simulink model "ProcessNetworkSimulation"  (R2015b)
settings: Solver=VariableStepAuto  StartTime=0.0  StopTime=1000.0  RelTol=1e-3
libraries: simulink x1, simeventslib x1
(part 8 of 21)

== system ProcessNetworkSimulation/Process_4 ==
  IN_Job : PathCombiner  NumberInputPorts=42
  OUT_Job : OutputSwitch  NumberOutputPorts=37  SwitchingCriterion=From attribute  AttributeName=outputFlowNode
  Process : Subsystem
  IN_Job_1 : PMIOPort  Port=1  Side=Left
  IN_Job_2 : PMIOPort  Port=2  Side=Left
  IN_Job_3 : PMIOPort  Port=3  Side=Left
  IN_Job_4 : PMIOPort  Port=4  Side=Left
  IN_Job_5 : PMIOPort  Port=5  Side=Left
  IN_Job_6 : PMIOPort  Port=6  Side=Left
  IN_Job_7 : PMIOPort  Port=7  Side=Left
  IN_Job_8 : PMIOPort  Port=8  Side=Left
  IN_Job_9 : PMIOPort  Port=9  Side=Left
  IN_Job_10 : PMIOPort  Port=10  Side=Left
  IN_Job_11 : PMIOPort  Port=11  Side=Left
  IN_Job_12 : PMIOPort  Port=12  Side=Left
  IN_Job_13 : PMIOPort  Port=13  Side=Left
  IN_Job_14 : PMIOPort  Port=14  Side=Left
  IN_Job_15 : PMIOPort  Port=15  Side=Left
  IN_Job_16 : PMIOPort  Port=16  Side=Left
  IN_Job_17 : PMIOPort  Port=17  Side=Left
  IN_Job_18 : PMIOPort  Port=18  Side=Left
  IN_Job_19 : PMIOPort  Port=19  Side=Left
  IN_Job_20 : PMIOPort  Port=20  Side=Left
  IN_Job_21 : PMIOPort  Port=21  Side=Left
  IN_Job_22 : PMIOPort  Port=22  Side=Left
  IN_Job_23 : PMIOPort  Port=23  Side=Left
  IN_Job_24 : PMIOPort  Port=24  Side=Left
  IN_Job_25 : PMIOPort  Port=25  Side=Left
  IN_Job_26 : PMIOPort  Port=26  Side=Left
  IN_Job_27 : PMIOPort  Port=27  Side=Left
  IN_Job_28 : PMIOPort  Port=28  Side=Left
  IN_Job_29 : PMIOPort  Port=29  Side=Left
  IN_Job_30 : PMIOPort  Port=30  Side=Left
  IN_Job_31 : PMIOPort  Port=31  Side=Left
  IN_Job_32 : PMIOPort  Port=32  Side=Left
  IN_Job_33 : PMIOPort  Port=33  Side=Left
  IN_Job_34 : PMIOPort  Port=34  Side=Left
  IN_Job_35 : PMIOPort  Port=35  Side=Left
  IN_Job_36 : PMIOPort  Port=36  Side=Left
  IN_Job_37 : PMIOPort  Port=37  Side=Left
  IN_Job_38 : PMIOPort  Port=38  Side=Left
  IN_Job_39 : PMIOPort  Port=39  Side=Left
  IN_Job_40 : PMIOPort  Port=40  Side=Left
  IN_Job_41 : PMIOPort  Port=41  Side=Left
  IN_Job_42 : PMIOPort  Port=42  Side=Left
  OUT_Job_1 : PMIOPort  Port=43  Side=Right
  OUT_Job_2 : PMIOPort  Port=44  Side=Right
  OUT_Job_3 : PMIOPort  Port=45  Side=Right
  OUT_Job_4 : PMIOPort  Port=46  Side=Right
  OUT_Job_5 : PMIOPort  Port=47  Side=Right
  OUT_Job_6 : PMIOPort  Port=48  Side=Right
  OUT_Job_7 : PMIOPort  Port=49  Side=Right
  OUT_Job_8 : PMIOPort  Port=50  Side=Right
  OUT_Job_9 : PMIOPort  Port=51  Side=Right
  OUT_Job_10 : PMIOPort  Port=52  Side=Right
  OUT_Job_11 : PMIOPort  Port=53  Side=Right
  OUT_Job_12 : PMIOPort  Port=54  Side=Right
  OUT_Job_13 : PMIOPort  Port=55  Side=Right
  OUT_Job_14 : PMIOPort  Port=56  Side=Right
  OUT_Job_15 : PMIOPort  Port=57  Side=Right
  OUT_Job_16 : PMIOPort  Port=58  Side=Right
  OUT_Job_17 : PMIOPort  Port=59  Side=Right
  OUT_Job_18 : PMIOPort  Port=60  Side=Right
  OUT_Job_19 : PMIOPort  Port=61  Side=Right
  OUT_Job_20 : PMIOPort  Port=62  Side=Right
  OUT_Job_21 : PMIOPort  Port=63  Side=Right
  OUT_Job_22 : PMIOPort  Port=64  Side=Right
  OUT_Job_23 : PMIOPort  Port=65  Side=Right
  OUT_Job_24 : PMIOPort  Port=66  Side=Right
  OUT_Job_25 : PMIOPort  Port=67  Side=Right
  OUT_Job_26 : PMIOPort  Port=68  Side=Right
  OUT_Job_27 : PMIOPort  Port=69  Side=Right
  OUT_Job_28 : PMIOPort  Port=70  Side=Right
  OUT_Job_29 : PMIOPort  Port=71  Side=Right
  OUT_Job_30 : PMIOPort  Port=72  Side=Right
  OUT_Job_31 : PMIOPort  Port=73  Side=Right
  OUT_Job_32 : PMIOPort  Port=74  Side=Right
  OUT_Job_33 : PMIOPort  Port=75  Side=Right
  OUT_Job_34 : PMIOPort  Port=76  Side=Right
  OUT_Job_35 : PMIOPort  Port=77  Side=Right
  OUT_Job_36 : PMIOPort  Port=78  Side=Right
  OUT_Job_37 : PMIOPort  Port=79  Side=Right
  connections:
  OUT_Job/LConn1 -- Process/RConn1
  IN_Job/RConn1 -- Process/LConn1
  IN_Job/LConn1 -- IN_Job_1/RConn1
  IN_Job/LConn2 -- IN_Job_2/RConn1
  IN_Job/LConn3 -- IN_Job_3/RConn1
  IN_Job/LConn4 -- IN_Job_4/RConn1
  IN_Job/LConn5 -- IN_Job_5/RConn1
  IN_Job/LConn6 -- IN_Job_6/RConn1
  IN_Job/LConn7 -- IN_Job_7/RConn1
  IN_Job/LConn8 -- IN_Job_8/RConn1
  IN_Job/LConn9 -- IN_Job_9/RConn1
  IN_Job/LConn10 -- IN_Job_10/RConn1
  IN_Job/LConn11 -- IN_Job_11/RConn1
  IN_Job/LConn12 -- IN_Job_12/RConn1
  IN_Job/LConn13 -- IN_Job_13/RConn1
  IN_Job/LConn14 -- IN_Job_14/RConn1
  IN_Job/LConn15 -- IN_Job_15/RConn1
  IN_Job/LConn16 -- IN_Job_16/RConn1
  IN_Job/LConn17 -- IN_Job_17/RConn1
  IN_Job/LConn18 -- IN_Job_18/RConn1
  IN_Job/LConn19 -- IN_Job_19/RConn1
  IN_Job/LConn20 -- IN_Job_20/RConn1
  IN_Job/LConn21 -- IN_Job_21/RConn1
  IN_Job/LConn22 -- IN_Job_22/RConn1
  IN_Job/LConn23 -- IN_Job_23/RConn1
  IN_Job/LConn24 -- IN_Job_24/RConn1
  IN_Job/LConn25 -- IN_Job_25/RConn1
  IN_Job/LConn26 -- IN_Job_26/RConn1
  IN_Job/LConn27 -- IN_Job_27/RConn1
  IN_Job/LConn28 -- IN_Job_28/RConn1
  IN_Job/LConn29 -- IN_Job_29/RConn1
  IN_Job/LConn30 -- IN_Job_30/RConn1
  IN_Job/LConn31 -- IN_Job_31/RConn1
  IN_Job/LConn32 -- IN_Job_32/RConn1
  IN_Job/LConn33 -- IN_Job_33/RConn1
  IN_Job/LConn34 -- IN_Job_34/RConn1
  IN_Job/LConn35 -- IN_Job_35/RConn1
  IN_Job/LConn36 -- IN_Job_36/RConn1
  IN_Job/LConn37 -- IN_Job_37/RConn1
  IN_Job/LConn38 -- IN_Job_38/RConn1
  IN_Job/LConn39 -- IN_Job_39/RConn1
  IN_Job/LConn40 -- IN_Job_40/RConn1
  IN_Job/LConn41 -- IN_Job_41/RConn1
  IN_Job/LConn42 -- IN_Job_42/RConn1
  OUT_Job/RConn1 -- OUT_Job_1/RConn1
  OUT_Job/RConn2 -- OUT_Job_2/RConn1
  OUT_Job/RConn3 -- OUT_Job_3/RConn1
  OUT_Job/RConn4 -- OUT_Job_4/RConn1
  OUT_Job/RConn5 -- OUT_Job_5/RConn1
  OUT_Job/RConn6 -- OUT_Job_6/RConn1
  OUT_Job/RConn7 -- OUT_Job_7/RConn1
  OUT_Job/RConn8 -- OUT_Job_8/RConn1
  OUT_Job/RConn9 -- OUT_Job_9/RConn1
  OUT_Job/RConn10 -- OUT_Job_10/RConn1
  OUT_Job/RConn11 -- OUT_Job_11/RConn1
  OUT_Job/RConn12 -- OUT_Job_12/RConn1
  OUT_Job/RConn13 -- OUT_Job_13/RConn1
  OUT_Job/RConn14 -- OUT_Job_14/RConn1
  OUT_Job/RConn15 -- OUT_Job_15/RConn1
  OUT_Job/RConn16 -- OUT_Job_16/RConn1
  OUT_Job/RConn17 -- OUT_Job_17/RConn1
  OUT_Job/RConn18 -- OUT_Job_18/RConn1
  OUT_Job/RConn19 -- OUT_Job_19/RConn1
  OUT_Job/RConn20 -- OUT_Job_20/RConn1
  OUT_Job/RConn21 -- OUT_Job_21/RConn1
  OUT_Job/RConn22 -- OUT_Job_22/RConn1
  OUT_Job/RConn23 -- OUT_Job_23/RConn1
  OUT_Job/RConn24 -- OUT_Job_24/RConn1
  OUT_Job/RConn25 -- OUT_Job_25/RConn1
  OUT_Job/RConn26 -- OUT_Job_26/RConn1
  OUT_Job/RConn27 -- OUT_Job_27/RConn1
  OUT_Job/RConn28 -- OUT_Job_28/RConn1
  OUT_Job/RConn29 -- OUT_Job_29/RConn1
  OUT_Job/RConn30 -- OUT_Job_30/RConn1
  OUT_Job/RConn31 -- OUT_Job_31/RConn1
  OUT_Job/RConn32 -- OUT_Job_32/RConn1
  OUT_Job/RConn33 -- OUT_Job_33/RConn1
  OUT_Job/RConn34 -- OUT_Job_34/RConn1
  OUT_Job/RConn35 -- OUT_Job_35/RConn1
  OUT_Job/RConn36 -- OUT_Job_36/RConn1
  OUT_Job/RConn37 -- OUT_Job_37/RConn1

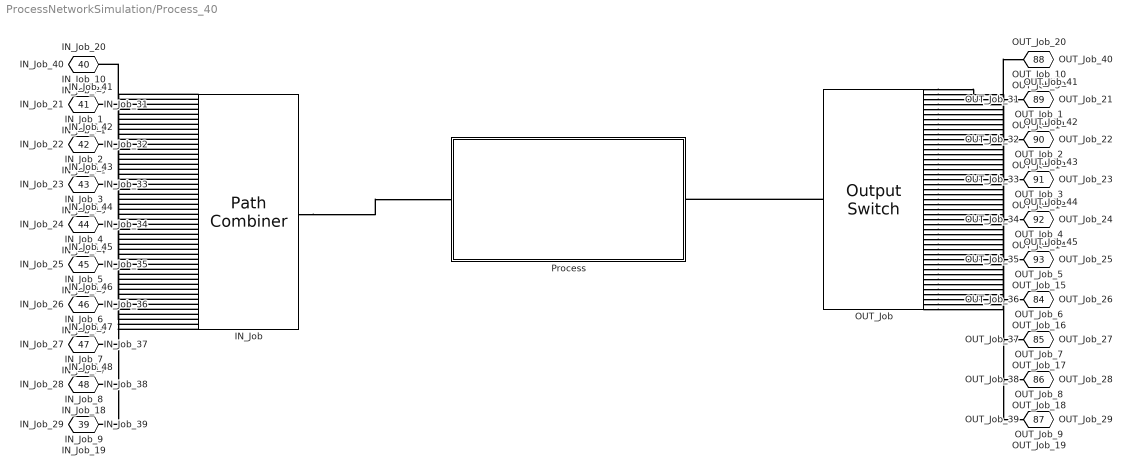
== system ProcessNetworkSimulation/Process_40 ==
  IN_Job : PathCombiner  NumberInputPorts=48
  OUT_Job : OutputSwitch  NumberOutputPorts=45  SwitchingCriterion=From attribute  AttributeName=outputFlowNode
  Process : Subsystem
  IN_Job_1 : PMIOPort  Port=1  Side=Left
  IN_Job_2 : PMIOPort  Port=2  Side=Left
  IN_Job_3 : PMIOPort  Port=3  Side=Left
  IN_Job_4 : PMIOPort  Port=4  Side=Left
  IN_Job_5 : PMIOPort  Port=5  Side=Left
  IN_Job_6 : PMIOPort  Port=6  Side=Left
  IN_Job_7 : PMIOPort  Port=7  Side=Left
  IN_Job_8 : PMIOPort  Port=8  Side=Left
  IN_Job_9 : PMIOPort  Port=9  Side=Left
  IN_Job_10 : PMIOPort  Port=10  Side=Left
  IN_Job_11 : PMIOPort  Port=11  Side=Left
  IN_Job_12 : PMIOPort  Port=12  Side=Left
  IN_Job_13 : PMIOPort  Port=13  Side=Left
  IN_Job_14 : PMIOPort  Port=14  Side=Left
  IN_Job_15 : PMIOPort  Port=15  Side=Left
  IN_Job_16 : PMIOPort  Port=16  Side=Left
  IN_Job_17 : PMIOPort  Port=17  Side=Left
  IN_Job_18 : PMIOPort  Port=18  Side=Left
  IN_Job_19 : PMIOPort  Port=19  Side=Left
  IN_Job_20 : PMIOPort  Port=20  Side=Left
  IN_Job_21 : PMIOPort  Port=21  Side=Left
  IN_Job_22 : PMIOPort  Port=22  Side=Left
  IN_Job_23 : PMIOPort  Port=23  Side=Left
  IN_Job_24 : PMIOPort  Port=24  Side=Left
  IN_Job_25 : PMIOPort  Port=25  Side=Left
  IN_Job_26 : PMIOPort  Port=26  Side=Left
  IN_Job_27 : PMIOPort  Port=27  Side=Left
  IN_Job_28 : PMIOPort  Port=28  Side=Left
  IN_Job_29 : PMIOPort  Port=29  Side=Left
  IN_Job_30 : PMIOPort  Port=30  Side=Left
  IN_Job_31 : PMIOPort  Port=31  Side=Left
  IN_Job_32 : PMIOPort  Port=32  Side=Left
  IN_Job_33 : PMIOPort  Port=33  Side=Left
  IN_Job_34 : PMIOPort  Port=34  Side=Left
  IN_Job_35 : PMIOPort  Port=35  Side=Left
  IN_Job_36 : PMIOPort  Port=36  Side=Left
  IN_Job_37 : PMIOPort  Port=37  Side=Left
  IN_Job_38 : PMIOPort  Port=38  Side=Left
  IN_Job_39 : PMIOPort  Port=39  Side=Left
  IN_Job_40 : PMIOPort  Port=40  Side=Left
  IN_Job_41 : PMIOPort  Port=41  Side=Left
  IN_Job_42 : PMIOPort  Port=42  Side=Left
  IN_Job_43 : PMIOPort  Port=43  Side=Left
  IN_Job_44 : PMIOPort  Port=44  Side=Left
  IN_Job_45 : PMIOPort  Port=45  Side=Left
  IN_Job_46 : PMIOPort  Port=46  Side=Left
  IN_Job_47 : PMIOPort  Port=47  Side=Left
  IN_Job_48 : PMIOPort  Port=48  Side=Left
  OUT_Job_1 : PMIOPort  Port=49  Side=Right
  OUT_Job_2 : PMIOPort  Port=50  Side=Right
  OUT_Job_3 : PMIOPort  Port=51  Side=Right
  OUT_Job_4 : PMIOPort  Port=52  Side=Right
  OUT_Job_5 : PMIOPort  Port=53  Side=Right
  OUT_Job_6 : PMIOPort  Port=54  Side=Right
  OUT_Job_7 : PMIOPort  Port=55  Side=Right
  OUT_Job_8 : PMIOPort  Port=56  Side=Right
  OUT_Job_9 : PMIOPort  Port=57  Side=Right
  OUT_Job_10 : PMIOPort  Port=58  Side=Right
  OUT_Job_11 : PMIOPort  Port=59  Side=Right
  OUT_Job_12 : PMIOPort  Port=60  Side=Right
  OUT_Job_13 : PMIOPort  Port=61  Side=Right
  OUT_Job_14 : PMIOPort  Port=62  Side=Right
  OUT_Job_15 : PMIOPort  Port=63  Side=Right
  OUT_Job_16 : PMIOPort  Port=64  Side=Right
  OUT_Job_17 : PMIOPort  Port=65  Side=Right
  OUT_Job_18 : PMIOPort  Port=66  Side=Right
  OUT_Job_19 : PMIOPort  Port=67  Side=Right
  OUT_Job_20 : PMIOPort  Port=68  Side=Right
  OUT_Job_21 : PMIOPort  Port=69  Side=Right
  OUT_Job_22 : PMIOPort  Port=70  Side=Right
  OUT_Job_23 : PMIOPort  Port=71  Side=Right
  OUT_Job_24 : PMIOPort  Port=72  Side=Right
  OUT_Job_25 : PMIOPort  Port=73  Side=Right
  OUT_Job_26 : PMIOPort  Port=74  Side=Right
  OUT_Job_27 : PMIOPort  Port=75  Side=Right
  OUT_Job_28 : PMIOPort  Port=76  Side=Right
  OUT_Job_29 : PMIOPort  Port=77  Side=Right
  OUT_Job_30 : PMIOPort  Port=78  Side=Right
  OUT_Job_31 : PMIOPort  Port=79  Side=Right
  OUT_Job_32 : PMIOPort  Port=80  Side=Right
  OUT_Job_33 : PMIOPort  Port=81  Side=Right
  OUT_Job_34 : PMIOPort  Port=82  Side=Right
  OUT_Job_35 : PMIOPort  Port=83  Side=Right
  OUT_Job_36 : PMIOPort  Port=84  Side=Right
  OUT_Job_37 : PMIOPort  Port=85  Side=Right
  OUT_Job_38 : PMIOPort  Port=86  Side=Right
  OUT_Job_39 : PMIOPort  Port=87  Side=Right
  OUT_Job_40 : PMIOPort  Port=88  Side=Right
  OUT_Job_41 : PMIOPort  Port=89  Side=Right
  OUT_Job_42 : PMIOPort  Port=90  Side=Right
  OUT_Job_43 : PMIOPort  Port=91  Side=Right
  OUT_Job_44 : PMIOPort  Port=92  Side=Right
  OUT_Job_45 : PMIOPort  Port=93  Side=Right
  connections:
  OUT_Job/LConn1 -- Process/RConn1
  IN_Job/RConn1 -- Process/LConn1
  IN_Job/LConn1 -- IN_Job_1/RConn1
  IN_Job/LConn2 -- IN_Job_2/RConn1
  IN_Job/LConn3 -- IN_Job_3/RConn1
  IN_Job/LConn4 -- IN_Job_4/RConn1
  IN_Job/LConn5 -- IN_Job_5/RConn1
  IN_Job/LConn6 -- IN_Job_6/RConn1
  IN_Job/LConn7 -- IN_Job_7/RConn1
  IN_Job/LConn8 -- IN_Job_8/RConn1
  IN_Job/LConn9 -- IN_Job_9/RConn1
  IN_Job/LConn10 -- IN_Job_10/RConn1
  IN_Job/LConn11 -- IN_Job_11/RConn1
  IN_Job/LConn12 -- IN_Job_12/RConn1
  IN_Job/LConn13 -- IN_Job_13/RConn1
  IN_Job/LConn14 -- IN_Job_14/RConn1
  IN_Job/LConn15 -- IN_Job_15/RConn1
  IN_Job/LConn16 -- IN_Job_16/RConn1
  IN_Job/LConn17 -- IN_Job_17/RConn1
  IN_Job/LConn18 -- IN_Job_18/RConn1
  IN_Job/LConn19 -- IN_Job_19/RConn1
  IN_Job/LConn20 -- IN_Job_20/RConn1
  IN_Job/LConn21 -- IN_Job_21/RConn1
  IN_Job/LConn22 -- IN_Job_22/RConn1
  IN_Job/LConn23 -- IN_Job_23/RConn1
  IN_Job/LConn24 -- IN_Job_24/RConn1
  IN_Job/LConn25 -- IN_Job_25/RConn1
  IN_Job/LConn26 -- IN_Job_26/RConn1
  IN_Job/LConn27 -- IN_Job_27/RConn1
  IN_Job/LConn28 -- IN_Job_28/RConn1
  IN_Job/LConn29 -- IN_Job_29/RConn1
  IN_Job/LConn30 -- IN_Job_30/RConn1
  IN_Job/LConn31 -- IN_Job_31/RConn1
  IN_Job/LConn32 -- IN_Job_32/RConn1
  IN_Job/LConn33 -- IN_Job_33/RConn1
  IN_Job/LConn34 -- IN_Job_34/RConn1
  IN_Job/LConn35 -- IN_Job_35/RConn1
  IN_Job/LConn36 -- IN_Job_36/RConn1
  IN_Job/LConn37 -- IN_Job_37/RConn1
  IN_Job/LConn38 -- IN_Job_38/RConn1
  IN_Job/LConn39 -- IN_Job_39/RConn1
  IN_Job/LConn40 -- IN_Job_40/RConn1
  IN_Job/LConn41 -- IN_Job_41/RConn1
  IN_Job/LConn42 -- IN_Job_42/RConn1
  IN_Job/LConn43 -- IN_Job_43/RConn1
  IN_Job/LConn44 -- IN_Job_44/RConn1
  IN_Job/LConn45 -- IN_Job_45/RConn1
  IN_Job/LConn46 -- IN_Job_46/RConn1
  IN_Job/LConn47 -- IN_Job_47/RConn1
  IN_Job/LConn48 -- IN_Job_48/RConn1
  OUT_Job/RConn1 -- OUT_Job_1/RConn1
  OUT_Job/RConn2 -- OUT_Job_2/RConn1
  OUT_Job/RConn3 -- OUT_Job_3/RConn1
  OUT_Job/RConn4 -- OUT_Job_4/RConn1
  OUT_Job/RConn5 -- OUT_Job_5/RConn1
  OUT_Job/RConn6 -- OUT_Job_6/RConn1
  OUT_Job/RConn7 -- OUT_Job_7/RConn1
  OUT_Job/RConn8 -- OUT_Job_8/RConn1
  OUT_Job/RConn9 -- OUT_Job_9/RConn1
  OUT_Job/RConn10 -- OUT_Job_10/RConn1
  OUT_Job/RConn11 -- OUT_Job_11/RConn1
  OUT_Job/RConn12 -- OUT_Job_12/RConn1
  OUT_Job/RConn13 -- OUT_Job_13/RConn1
  OUT_Job/RConn14 -- OUT_Job_14/RConn1
  OUT_Job/RConn15 -- OUT_Job_15/RConn1
  OUT_Job/RConn16 -- OUT_Job_16/RConn1
  OUT_Job/RConn17 -- OUT_Job_17/RConn1
  OUT_Job/RConn18 -- OUT_Job_18/RConn1
  OUT_Job/RConn19 -- OUT_Job_19/RConn1
  OUT_Job/RConn20 -- OUT_Job_20/RConn1
  OUT_Job/RConn21 -- OUT_Job_21/RConn1
  OUT_Job/RConn22 -- OUT_Job_22/RConn1
  OUT_Job/RConn23 -- OUT_Job_23/RConn1
  OUT_Job/RConn24 -- OUT_Job_24/RConn1
  OUT_Job/RConn25 -- OUT_Job_25/RConn1
  OUT_Job/RConn26 -- OUT_Job_26/RConn1
  OUT_Job/RConn27 -- OUT_Job_27/RConn1
  OUT_Job/RConn28 -- OUT_Job_28/RConn1
  OUT_Job/RConn29 -- OUT_Job_29/RConn1
  OUT_Job/RConn30 -- OUT_Job_30/RConn1
  OUT_Job/RConn31 -- OUT_Job_31/RConn1
  OUT_Job/RConn32 -- OUT_Job_32/RConn1
  OUT_Job/RConn33 -- OUT_Job_33/RConn1
  OUT_Job/RConn34 -- OUT_Job_34/RConn1
  OUT_Job/RConn35 -- OUT_Job_35/RConn1
  OUT_Job/RConn36 -- OUT_Job_36/RConn1
  OUT_Job/RConn37 -- OUT_Job_37/RConn1
  OUT_Job/RConn38 -- OUT_Job_38/RConn1
  OUT_Job/RConn39 -- OUT_Job_39/RConn1
  OUT_Job/RConn40 -- OUT_Job_40/RConn1
  OUT_Job/RConn41 -- OUT_Job_41/RConn1
  OUT_Job/RConn42 -- OUT_Job_42/RConn1
  OUT_Job/RConn43 -- OUT_Job_43/RConn1
  OUT_Job/RConn44 -- OUT_Job_44/RConn1
  OUT_Job/RConn45 -- OUT_Job_45/RConn1

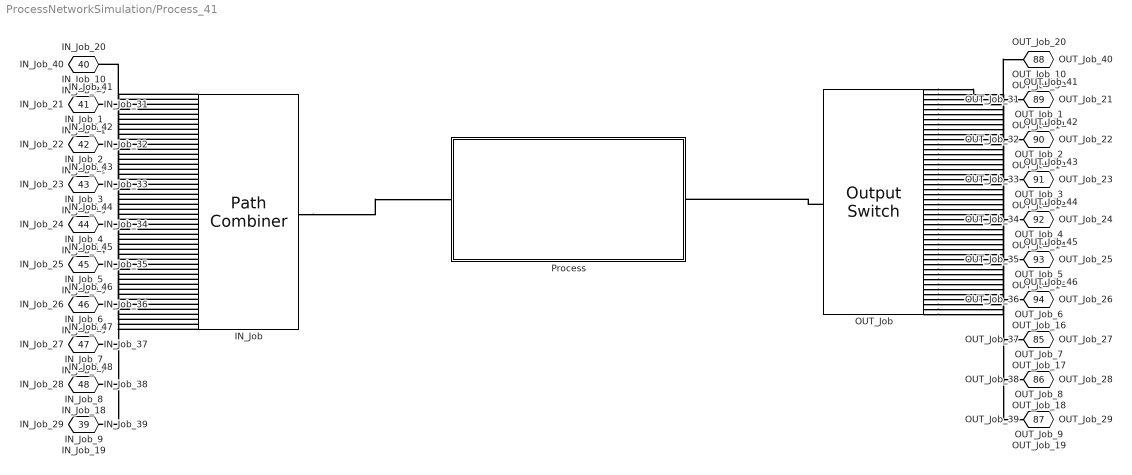
== system ProcessNetworkSimulation/Process_41 ==
  IN_Job : PathCombiner  NumberInputPorts=48
  OUT_Job : OutputSwitch  NumberOutputPorts=46  SwitchingCriterion=From attribute  AttributeName=outputFlowNode
  Process : Subsystem
  IN_Job_1 : PMIOPort  Port=1  Side=Left
  IN_Job_2 : PMIOPort  Port=2  Side=Left
  IN_Job_3 : PMIOPort  Port=3  Side=Left
  IN_Job_4 : PMIOPort  Port=4  Side=Left
  IN_Job_5 : PMIOPort  Port=5  Side=Left
  IN_Job_6 : PMIOPort  Port=6  Side=Left
  IN_Job_7 : PMIOPort  Port=7  Side=Left
  IN_Job_8 : PMIOPort  Port=8  Side=Left
  IN_Job_9 : PMIOPort  Port=9  Side=Left
  IN_Job_10 : PMIOPort  Port=10  Side=Left
  IN_Job_11 : PMIOPort  Port=11  Side=Left
  IN_Job_12 : PMIOPort  Port=12  Side=Left
  IN_Job_13 : PMIOPort  Port=13  Side=Left
  IN_Job_14 : PMIOPort  Port=14  Side=Left
  IN_Job_15 : PMIOPort  Port=15  Side=Left
  IN_Job_16 : PMIOPort  Port=16  Side=Left
  IN_Job_17 : PMIOPort  Port=17  Side=Left
  IN_Job_18 : PMIOPort  Port=18  Side=Left
  IN_Job_19 : PMIOPort  Port=19  Side=Left
  IN_Job_20 : PMIOPort  Port=20  Side=Left
  IN_Job_21 : PMIOPort  Port=21  Side=Left
  IN_Job_22 : PMIOPort  Port=22  Side=Left
  IN_Job_23 : PMIOPort  Port=23  Side=Left
  IN_Job_24 : PMIOPort  Port=24  Side=Left
  IN_Job_25 : PMIOPort  Port=25  Side=Left
  IN_Job_26 : PMIOPort  Port=26  Side=Left
  IN_Job_27 : PMIOPort  Port=27  Side=Left
  IN_Job_28 : PMIOPort  Port=28  Side=Left
  IN_Job_29 : PMIOPort  Port=29  Side=Left
  IN_Job_30 : PMIOPort  Port=30  Side=Left
  IN_Job_31 : PMIOPort  Port=31  Side=Left
  IN_Job_32 : PMIOPort  Port=32  Side=Left
  IN_Job_33 : PMIOPort  Port=33  Side=Left
  IN_Job_34 : PMIOPort  Port=34  Side=Left
  IN_Job_35 : PMIOPort  Port=35  Side=Left
  IN_Job_36 : PMIOPort  Port=36  Side=Left
  IN_Job_37 : PMIOPort  Port=37  Side=Left
  IN_Job_38 : PMIOPort  Port=38  Side=Left
  IN_Job_39 : PMIOPort  Port=39  Side=Left
  IN_Job_40 : PMIOPort  Port=40  Side=Left
  IN_Job_41 : PMIOPort  Port=41  Side=Left
  IN_Job_42 : PMIOPort  Port=42  Side=Left
  IN_Job_43 : PMIOPort  Port=43  Side=Left
  IN_Job_44 : PMIOPort  Port=44  Side=Left
  IN_Job_45 : PMIOPort  Port=45  Side=Left
  IN_Job_46 : PMIOPort  Port=46  Side=Left
  IN_Job_47 : PMIOPort  Port=47  Side=Left
  IN_Job_48 : PMIOPort  Port=48  Side=Left
  OUT_Job_1 : PMIOPort  Port=49  Side=Right
  OUT_Job_2 : PMIOPort  Port=50  Side=Right
  OUT_Job_3 : PMIOPort  Port=51  Side=Right
  OUT_Job_4 : PMIOPort  Port=52  Side=Right
  OUT_Job_5 : PMIOPort  Port=53  Side=Right
  OUT_Job_6 : PMIOPort  Port=54  Side=Right
  OUT_Job_7 : PMIOPort  Port=55  Side=Right
  OUT_Job_8 : PMIOPort  Port=56  Side=Right
  OUT_Job_9 : PMIOPort  Port=57  Side=Right
  OUT_Job_10 : PMIOPort  Port=58  Side=Right
  OUT_Job_11 : PMIOPort  Port=59  Side=Right
  OUT_Job_12 : PMIOPort  Port=60  Side=Right
  OUT_Job_13 : PMIOPort  Port=61  Side=Right
  OUT_Job_14 : PMIOPort  Port=62  Side=Right
  OUT_Job_15 : PMIOPort  Port=63  Side=Right
  OUT_Job_16 : PMIOPort  Port=64  Side=Right
  OUT_Job_17 : PMIOPort  Port=65  Side=Right
  OUT_Job_18 : PMIOPort  Port=66  Side=Right
  OUT_Job_19 : PMIOPort  Port=67  Side=Right
  OUT_Job_20 : PMIOPort  Port=68  Side=Right
  OUT_Job_21 : PMIOPort  Port=69  Side=Right
  OUT_Job_22 : PMIOPort  Port=70  Side=Right
  OUT_Job_23 : PMIOPort  Port=71  Side=Right
  OUT_Job_24 : PMIOPort  Port=72  Side=Right
  OUT_Job_25 : PMIOPort  Port=73  Side=Right
  OUT_Job_26 : PMIOPort  Port=74  Side=Right
  OUT_Job_27 : PMIOPort  Port=75  Side=Right
  OUT_Job_28 : PMIOPort  Port=76  Side=Right
  OUT_Job_29 : PMIOPort  Port=77  Side=Right
  OUT_Job_30 : PMIOPort  Port=78  Side=Right
  OUT_Job_31 : PMIOPort  Port=79  Side=Right
  OUT_Job_32 : PMIOPort  Port=80  Side=Right
  OUT_Job_33 : PMIOPort  Port=81  Side=Right
  OUT_Job_34 : PMIOPort  Port=82  Side=Right
  OUT_Job_35 : PMIOPort  Port=83  Side=Right
  OUT_Job_36 : PMIOPort  Port=84  Side=Right
  OUT_Job_37 : PMIOPort  Port=85  Side=Right
  OUT_Job_38 : PMIOPort  Port=86  Side=Right
  OUT_Job_39 : PMIOPort  Port=87  Side=Right
  OUT_Job_40 : PMIOPort  Port=88  Side=Right
  OUT_Job_41 : PMIOPort  Port=89  Side=Right
  OUT_Job_42 : PMIOPort  Port=90  Side=Right
  OUT_Job_43 : PMIOPort  Port=91  Side=Right
  OUT_Job_44 : PMIOPort  Port=92  Side=Right
  OUT_Job_45 : PMIOPort  Port=93  Side=Right
  OUT_Job_46 : PMIOPort  Port=94  Side=Right
  connections:
  OUT_Job/LConn1 -- Process/RConn1
  IN_Job/RConn1 -- Process/LConn1
  IN_Job/LConn1 -- IN_Job_1/RConn1
  IN_Job/LConn2 -- IN_Job_2/RConn1
  IN_Job/LConn3 -- IN_Job_3/RConn1
  IN_Job/LConn4 -- IN_Job_4/RConn1
  IN_Job/LConn5 -- IN_Job_5/RConn1
  IN_Job/LConn6 -- IN_Job_6/RConn1
  IN_Job/LConn7 -- IN_Job_7/RConn1
  IN_Job/LConn8 -- IN_Job_8/RConn1
  IN_Job/LConn9 -- IN_Job_9/RConn1
  IN_Job/LConn10 -- IN_Job_10/RConn1
  IN_Job/LConn11 -- IN_Job_11/RConn1
  IN_Job/LConn12 -- IN_Job_12/RConn1
  IN_Job/LConn13 -- IN_Job_13/RConn1
  IN_Job/LConn14 -- IN_Job_14/RConn1
  IN_Job/LConn15 -- IN_Job_15/RConn1
  IN_Job/LConn16 -- IN_Job_16/RConn1
  IN_Job/LConn17 -- IN_Job_17/RConn1
  IN_Job/LConn18 -- IN_Job_18/RConn1
  IN_Job/LConn19 -- IN_Job_19/RConn1
  IN_Job/LConn20 -- IN_Job_20/RConn1
  IN_Job/LConn21 -- IN_Job_21/RConn1
  IN_Job/LConn22 -- IN_Job_22/RConn1
  IN_Job/LConn23 -- IN_Job_23/RConn1
  IN_Job/LConn24 -- IN_Job_24/RConn1
  IN_Job/LConn25 -- IN_Job_25/RConn1
  IN_Job/LConn26 -- IN_Job_26/RConn1
  IN_Job/LConn27 -- IN_Job_27/RConn1
  IN_Job/LConn28 -- IN_Job_28/RConn1
  IN_Job/LConn29 -- IN_Job_29/RConn1
  IN_Job/LConn30 -- IN_Job_30/RConn1
  IN_Job/LConn31 -- IN_Job_31/RConn1
  IN_Job/LConn32 -- IN_Job_32/RConn1
  IN_Job/LConn33 -- IN_Job_33/RConn1
  IN_Job/LConn34 -- IN_Job_34/RConn1
  IN_Job/LConn35 -- IN_Job_35/RConn1
  IN_Job/LConn36 -- IN_Job_36/RConn1
  IN_Job/LConn37 -- IN_Job_37/RConn1
  IN_Job/LConn38 -- IN_Job_38/RConn1
  IN_Job/LConn39 -- IN_Job_39/RConn1
  IN_Job/LConn40 -- IN_Job_40/RConn1
  IN_Job/LConn41 -- IN_Job_41/RConn1
  IN_Job/LConn42 -- IN_Job_42/RConn1
  IN_Job/LConn43 -- IN_Job_43/RConn1
  IN_Job/LConn44 -- IN_Job_44/RConn1
  IN_Job/LConn45 -- IN_Job_45/RConn1
  IN_Job/LConn46 -- IN_Job_46/RConn1
  IN_Job/LConn47 -- IN_Job_47/RConn1
  IN_Job/LConn48 -- IN_Job_48/RConn1
  OUT_Job/RConn1 -- OUT_Job_1/RConn1
  OUT_Job/RConn2 -- OUT_Job_2/RConn1
  OUT_Job/RConn3 -- OUT_Job_3/RConn1
  OUT_Job/RConn4 -- OUT_Job_4/RConn1
  OUT_Job/RConn5 -- OUT_Job_5/RConn1
  OUT_Job/RConn6 -- OUT_Job_6/RConn1
  OUT_Job/RConn7 -- OUT_Job_7/RConn1
  OUT_Job/RConn8 -- OUT_Job_8/RConn1
  OUT_Job/RConn9 -- OUT_Job_9/RConn1
  OUT_Job/RConn10 -- OUT_Job_10/RConn1
  OUT_Job/RConn11 -- OUT_Job_11/RConn1
  OUT_Job/RConn12 -- OUT_Job_12/RConn1
  OUT_Job/RConn13 -- OUT_Job_13/RConn1
  OUT_Job/RConn14 -- OUT_Job_14/RConn1
  OUT_Job/RConn15 -- OUT_Job_15/RConn1
  OUT_Job/RConn16 -- OUT_Job_16/RConn1
  OUT_Job/RConn17 -- OUT_Job_17/RConn1
  OUT_Job/RConn18 -- OUT_Job_18/RConn1
  OUT_Job/RConn19 -- OUT_Job_19/RConn1
  OUT_Job/RConn20 -- OUT_Job_20/RConn1
  OUT_Job/RConn21 -- OUT_Job_21/RConn1
  OUT_Job/RConn22 -- OUT_Job_22/RConn1
  OUT_Job/RConn23 -- OUT_Job_23/RConn1
  OUT_Job/RConn24 -- OUT_Job_24/RConn1
  OUT_Job/RConn25 -- OUT_Job_25/RConn1
  OUT_Job/RConn26 -- OUT_Job_26/RConn1
  OUT_Job/RConn27 -- OUT_Job_27/RConn1
  OUT_Job/RConn28 -- OUT_Job_28/RConn1
  OUT_Job/RConn29 -- OUT_Job_29/RConn1
  OUT_Job/RConn30 -- OUT_Job_30/RConn1
  OUT_Job/RConn31 -- OUT_Job_31/RConn1
  OUT_Job/RConn32 -- OUT_Job_32/RConn1
  OUT_Job/RConn33 -- OUT_Job_33/RConn1
  OUT_Job/RConn34 -- OUT_Job_34/RConn1
  OUT_Job/RConn35 -- OUT_Job_35/RConn1
  OUT_Job/RConn36 -- OUT_Job_36/RConn1
  OUT_Job/RConn37 -- OUT_Job_37/RConn1
  OUT_Job/RConn38 -- OUT_Job_38/RConn1
  OUT_Job/RConn39 -- OUT_Job_39/RConn1
  OUT_Job/RConn40 -- OUT_Job_40/RConn1
  OUT_Job/RConn41 -- OUT_Job_41/RConn1
  OUT_Job/RConn42 -- OUT_Job_42/RConn1
  OUT_Job/RConn43 -- OUT_Job_43/RConn1
  OUT_Job/RConn44 -- OUT_Job_44/RConn1
  OUT_Job/RConn45 -- OUT_Job_45/RConn1
  OUT_Job/RConn46 -- OUT_Job_46/RConn1

== system ProcessNetworkSimulation/Process_42 ==
  IN_Job : PathCombiner  NumberInputPorts=34
  OUT_Job : OutputSwitch  NumberOutputPorts=34  SwitchingCriterion=From attribute  AttributeName=outputFlowNode
  Process : Subsystem
  IN_Job_1 : PMIOPort  Port=1  Side=Left
  IN_Job_2 : PMIOPort  Port=2  Side=Left
  IN_Job_3 : PMIOPort  Port=3  Side=Left
  IN_Job_4 : PMIOPort  Port=4  Side=Left
  IN_Job_5 : PMIOPort  Port=5  Side=Left
  IN_Job_6 : PMIOPort  Port=6  Side=Left
  IN_Job_7 : PMIOPort  Port=7  Side=Left
  IN_Job_8 : PMIOPort  Port=8  Side=Left
  IN_Job_9 : PMIOPort  Port=9  Side=Left
  IN_Job_10 : PMIOPort  Port=10  Side=Left
  IN_Job_11 : PMIOPort  Port=11  Side=Left
  IN_Job_12 : PMIOPort  Port=12  Side=Left
  IN_Job_13 : PMIOPort  Port=13  Side=Left
  IN_Job_14 : PMIOPort  Port=14  Side=Left
  IN_Job_15 : PMIOPort  Port=15  Side=Left
  IN_Job_16 : PMIOPort  Port=16  Side=Left
  IN_Job_17 : PMIOPort  Port=17  Side=Left
  IN_Job_18 : PMIOPort  Port=18  Side=Left
  IN_Job_19 : PMIOPort  Port=19  Side=Left
  IN_Job_20 : PMIOPort  Port=20  Side=Left
  IN_Job_21 : PMIOPort  Port=21  Side=Left
  IN_Job_22 : PMIOPort  Port=22  Side=Left
  IN_Job_23 : PMIOPort  Port=23  Side=Left
  IN_Job_24 : PMIOPort  Port=24  Side=Left
  IN_Job_25 : PMIOPort  Port=25  Side=Left
  IN_Job_26 : PMIOPort  Port=26  Side=Left
  IN_Job_27 : PMIOPort  Port=27  Side=Left
  IN_Job_28 : PMIOPort  Port=28  Side=Left
  IN_Job_29 : PMIOPort  Port=29  Side=Left
  IN_Job_30 : PMIOPort  Port=30  Side=Left
  IN_Job_31 : PMIOPort  Port=31  Side=Left
  IN_Job_32 : PMIOPort  Port=32  Side=Left
  IN_Job_33 : PMIOPort  Port=33  Side=Left
  IN_Job_34 : PMIOPort  Port=34  Side=Left
  OUT_Job_1 : PMIOPort  Port=35  Side=Right
  OUT_Job_2 : PMIOPort  Port=36  Side=Right
  OUT_Job_3 : PMIOPort  Port=37  Side=Right
  OUT_Job_4 : PMIOPort  Port=38  Side=Right
  OUT_Job_5 : PMIOPort  Port=39  Side=Right
  OUT_Job_6 : PMIOPort  Port=40  Side=Right
  OUT_Job_7 : PMIOPort  Port=41  Side=Right
  OUT_Job_8 : PMIOPort  Port=42  Side=Right
  OUT_Job_9 : PMIOPort  Port=43  Side=Right
  OUT_Job_10 : PMIOPort  Port=44  Side=Right
  OUT_Job_11 : PMIOPort  Port=45  Side=Right
  OUT_Job_12 : PMIOPort  Port=46  Side=Right
  OUT_Job_13 : PMIOPort  Port=47  Side=Right
  OUT_Job_14 : PMIOPort  Port=48  Side=Right
  OUT_Job_15 : PMIOPort  Port=49  Side=Right
  OUT_Job_16 : PMIOPort  Port=50  Side=Right
  OUT_Job_17 : PMIOPort  Port=51  Side=Right
  OUT_Job_18 : PMIOPort  Port=52  Side=Right
  OUT_Job_19 : PMIOPort  Port=53  Side=Right
  OUT_Job_20 : PMIOPort  Port=54  Side=Right
  OUT_Job_21 : PMIOPort  Port=55  Side=Right
  OUT_Job_22 : PMIOPort  Port=56  Side=Right
  OUT_Job_23 : PMIOPort  Port=57  Side=Right
  OUT_Job_24 : PMIOPort  Port=58  Side=Right
  OUT_Job_25 : PMIOPort  Port=59  Side=Right
  OUT_Job_26 : PMIOPort  Port=60  Side=Right
  OUT_Job_27 : PMIOPort  Port=61  Side=Right
  OUT_Job_28 : PMIOPort  Port=62  Side=Right
  OUT_Job_29 : PMIOPort  Port=63  Side=Right
  OUT_Job_30 : PMIOPort  Port=64  Side=Right
  OUT_Job_31 : PMIOPort  Port=65  Side=Right
  OUT_Job_32 : PMIOPort  Port=66  Side=Right
  OUT_Job_33 : PMIOPort  Port=67  Side=Right
  OUT_Job_34 : PMIOPort  Port=68  Side=Right
  connections:
  OUT_Job/LConn1 -- Process/RConn1
  IN_Job/RConn1 -- Process/LConn1
  IN_Job/LConn1 -- IN_Job_1/RConn1
  IN_Job/LConn2 -- IN_Job_2/RConn1
  IN_Job/LConn3 -- IN_Job_3/RConn1
  IN_Job/LConn4 -- IN_Job_4/RConn1
  IN_Job/LConn5 -- IN_Job_5/RConn1
  IN_Job/LConn6 -- IN_Job_6/RConn1
  IN_Job/LConn7 -- IN_Job_7/RConn1
  IN_Job/LConn8 -- IN_Job_8/RConn1
  IN_Job/LConn9 -- IN_Job_9/RConn1
  IN_Job/LConn10 -- IN_Job_10/RConn1
  IN_Job/LConn11 -- IN_Job_11/RConn1
  IN_Job/LConn12 -- IN_Job_12/RConn1
  IN_Job/LConn13 -- IN_Job_13/RConn1
  IN_Job/LConn14 -- IN_Job_14/RConn1
  IN_Job/LConn15 -- IN_Job_15/RConn1
  IN_Job/LConn16 -- IN_Job_16/RConn1
  IN_Job/LConn17 -- IN_Job_17/RConn1
  IN_Job/LConn18 -- IN_Job_18/RConn1
  IN_Job/LConn19 -- IN_Job_19/RConn1
  IN_Job/LConn20 -- IN_Job_20/RConn1
  IN_Job/LConn21 -- IN_Job_21/RConn1
  IN_Job/LConn22 -- IN_Job_22/RConn1
  IN_Job/LConn23 -- IN_Job_23/RConn1
  IN_Job/LConn24 -- IN_Job_24/RConn1
  IN_Job/LConn25 -- IN_Job_25/RConn1
  IN_Job/LConn26 -- IN_Job_26/RConn1
  IN_Job/LConn27 -- IN_Job_27/RConn1
  IN_Job/LConn28 -- IN_Job_28/RConn1
  IN_Job/LConn29 -- IN_Job_29/RConn1
  IN_Job/LConn30 -- IN_Job_30/RConn1
  IN_Job/LConn31 -- IN_Job_31/RConn1
  IN_Job/LConn32 -- IN_Job_32/RConn1
  IN_Job/LConn33 -- IN_Job_33/RConn1
  IN_Job/LConn34 -- IN_Job_34/RConn1
  OUT_Job/RConn1 -- OUT_Job_1/RConn1
  OUT_Job/RConn2 -- OUT_Job_2/RConn1
  OUT_Job/RConn3 -- OUT_Job_3/RConn1
  OUT_Job/RConn4 -- OUT_Job_4/RConn1
  OUT_Job/RConn5 -- OUT_Job_5/RConn1
  OUT_Job/RConn6 -- OUT_Job_6/RConn1
  OUT_Job/RConn7 -- OUT_Job_7/RConn1
  OUT_Job/RConn8 -- OUT_Job_8/RConn1
  OUT_Job/RConn9 -- OUT_Job_9/RConn1
  OUT_Job/RConn10 -- OUT_Job_10/RConn1
  OUT_Job/RConn11 -- OUT_Job_11/RConn1
  OUT_Job/RConn12 -- OUT_Job_12/RConn1
  OUT_Job/RConn13 -- OUT_Job_13/RConn1
  OUT_Job/RConn14 -- OUT_Job_14/RConn1
  OUT_Job/RConn15 -- OUT_Job_15/RConn1
  OUT_Job/RConn16 -- OUT_Job_16/RConn1
  OUT_Job/RConn17 -- OUT_Job_17/RConn1
  OUT_Job/RConn18 -- OUT_Job_18/RConn1
  OUT_Job/RConn19 -- OUT_Job_19/RConn1
  OUT_Job/RConn20 -- OUT_Job_20/RConn1
  OUT_Job/RConn21 -- OUT_Job_21/RConn1
  OUT_Job/RConn22 -- OUT_Job_22/RConn1
  OUT_Job/RConn23 -- OUT_Job_23/RConn1
  OUT_Job/RConn24 -- OUT_Job_24/RConn1
  OUT_Job/RConn25 -- OUT_Job_25/RConn1
  OUT_Job/RConn26 -- OUT_Job_26/RConn1
  OUT_Job/RConn27 -- OUT_Job_27/RConn1
  OUT_Job/RConn28 -- OUT_Job_28/RConn1
  OUT_Job/RConn29 -- OUT_Job_29/RConn1
  OUT_Job/RConn30 -- OUT_Job_30/RConn1
  OUT_Job/RConn31 -- OUT_Job_31/RConn1
  OUT_Job/RConn32 -- OUT_Job_32/RConn1
  OUT_Job/RConn33 -- OUT_Job_33/RConn1
  OUT_Job/RConn34 -- OUT_Job_34/RConn1

== system ProcessNetworkSimulation/Process_43 ==
  IN_Job : PathCombiner  NumberInputPorts=40
  OUT_Job : OutputSwitch  NumberOutputPorts=42  SwitchingCriterion=From attribute  AttributeName=outputFlowNode
  Process : Subsystem
  IN_Job_1 : PMIOPort  Port=1  Side=Left
  IN_Job_2 : PMIOPort  Port=2  Side=Left
  IN_Job_3 : PMIOPort  Port=3  Side=Left
  IN_Job_4 : PMIOPort  Port=4  Side=Left
  IN_Job_5 : PMIOPort  Port=5  Side=Left
  IN_Job_6 : PMIOPort  Port=6  Side=Left
  IN_Job_7 : PMIOPort  Port=7  Side=Left
  IN_Job_8 : PMIOPort  Port=8  Side=Left
  IN_Job_9 : PMIOPort  Port=9  Side=Left
  IN_Job_10 : PMIOPort  Port=10  Side=Left
  IN_Job_11 : PMIOPort  Port=11  Side=Left
  IN_Job_12 : PMIOPort  Port=12  Side=Left
  IN_Job_13 : PMIOPort  Port=13  Side=Left
  IN_Job_14 : PMIOPort  Port=14  Side=Left
  IN_Job_15 : PMIOPort  Port=15  Side=Left
  IN_Job_16 : PMIOPort  Port=16  Side=Left
  IN_Job_17 : PMIOPort  Port=17  Side=Left
  IN_Job_18 : PMIOPort  Port=18  Side=Left
  IN_Job_19 : PMIOPort  Port=19  Side=Left
  IN_Job_20 : PMIOPort  Port=20  Side=Left
  IN_Job_21 : PMIOPort  Port=21  Side=Left
  IN_Job_22 : PMIOPort  Port=22  Side=Left
  IN_Job_23 : PMIOPort  Port=23  Side=Left
  IN_Job_24 : PMIOPort  Port=24  Side=Left
  IN_Job_25 : PMIOPort  Port=25  Side=Left
  IN_Job_26 : PMIOPort  Port=26  Side=Left
  IN_Job_27 : PMIOPort  Port=27  Side=Left
  IN_Job_28 : PMIOPort  Port=28  Side=Left
  IN_Job_29 : PMIOPort  Port=29  Side=Left
  IN_Job_30 : PMIOPort  Port=30  Side=Left
  IN_Job_31 : PMIOPort  Port=31  Side=Left
  IN_Job_32 : PMIOPort  Port=32  Side=Left
  IN_Job_33 : PMIOPort  Port=33  Side=Left
  IN_Job_34 : PMIOPort  Port=34  Side=Left
  IN_Job_35 : PMIOPort  Port=35  Side=Left
  IN_Job_36 : PMIOPort  Port=36  Side=Left
  IN_Job_37 : PMIOPort  Port=37  Side=Left
  IN_Job_38 : PMIOPort  Port=38  Side=Left
  IN_Job_39 : PMIOPort  Port=39  Side=Left
  IN_Job_40 : PMIOPort  Port=40  Side=Left
  OUT_Job_1 : PMIOPort  Port=41  Side=Right
  OUT_Job_2 : PMIOPort  Port=42  Side=Right
  OUT_Job_3 : PMIOPort  Port=43  Side=Right
  OUT_Job_4 : PMIOPort  Port=44  Side=Right
  OUT_Job_5 : PMIOPort  Port=45  Side=Right
  OUT_Job_6 : PMIOPort  Port=46  Side=Right
  OUT_Job_7 : PMIOPort  Port=47  Side=Right
  OUT_Job_8 : PMIOPort  Port=48  Side=Right
  OUT_Job_9 : PMIOPort  Port=49  Side=Right
  OUT_Job_10 : PMIOPort  Port=50  Side=Right
  OUT_Job_11 : PMIOPort  Port=51  Side=Right
  OUT_Job_12 : PMIOPort  Port=52  Side=Right
  OUT_Job_13 : PMIOPort  Port=53  Side=Right
  OUT_Job_14 : PMIOPort  Port=54  Side=Right
  OUT_Job_15 : PMIOPort  Port=55  Side=Right
  OUT_Job_16 : PMIOPort  Port=56  Side=Right
  OUT_Job_17 : PMIOPort  Port=57  Side=Right
  OUT_Job_18 : PMIOPort  Port=58  Side=Right
  OUT_Job_19 : PMIOPort  Port=59  Side=Right
  OUT_Job_20 : PMIOPort  Port=60  Side=Right
  OUT_Job_21 : PMIOPort  Port=61  Side=Right
  OUT_Job_22 : PMIOPort  Port=62  Side=Right
  OUT_Job_23 : PMIOPort  Port=63  Side=Right
  OUT_Job_24 : PMIOPort  Port=64  Side=Right
  OUT_Job_25 : PMIOPort  Port=65  Side=Right
  OUT_Job_26 : PMIOPort  Port=66  Side=Right
  OUT_Job_27 : PMIOPort  Port=67  Side=Right
  OUT_Job_28 : PMIOPort  Port=68  Side=Right
  OUT_Job_29 : PMIOPort  Port=69  Side=Right
  OUT_Job_30 : PMIOPort  Port=70  Side=Right
  OUT_Job_31 : PMIOPort  Port=71  Side=Right
  OUT_Job_32 : PMIOPort  Port=72  Side=Right
  OUT_Job_33 : PMIOPort  Port=73  Side=Right
  OUT_Job_34 : PMIOPort  Port=74  Side=Right
  OUT_Job_35 : PMIOPort  Port=75  Side=Right
  OUT_Job_36 : PMIOPort  Port=76  Side=Right
  OUT_Job_37 : PMIOPort  Port=77  Side=Right
  OUT_Job_38 : PMIOPort  Port=78  Side=Right
  OUT_Job_39 : PMIOPort  Port=79  Side=Right
  OUT_Job_40 : PMIOPort  Port=80  Side=Right
  OUT_Job_41 : PMIOPort  Port=81  Side=Right
  OUT_Job_42 : PMIOPort  Port=82  Side=Right
  connections:
  OUT_Job/LConn1 -- Process/RConn1
  IN_Job/RConn1 -- Process/LConn1
  IN_Job/LConn1 -- IN_Job_1/RConn1
  IN_Job/LConn2 -- IN_Job_2/RConn1
  IN_Job/LConn3 -- IN_Job_3/RConn1
  IN_Job/LConn4 -- IN_Job_4/RConn1
  IN_Job/LConn5 -- IN_Job_5/RConn1
  IN_Job/LConn6 -- IN_Job_6/RConn1
  IN_Job/LConn7 -- IN_Job_7/RConn1
  IN_Job/LConn8 -- IN_Job_8/RConn1
  IN_Job/LConn9 -- IN_Job_9/RConn1
  IN_Job/LConn10 -- IN_Job_10/RConn1
  IN_Job/LConn11 -- IN_Job_11/RConn1
  IN_Job/LConn12 -- IN_Job_12/RConn1
  IN_Job/LConn13 -- IN_Job_13/RConn1
  IN_Job/LConn14 -- IN_Job_14/RConn1
  IN_Job/LConn15 -- IN_Job_15/RConn1
  IN_Job/LConn16 -- IN_Job_16/RConn1
  IN_Job/LConn17 -- IN_Job_17/RConn1
  IN_Job/LConn18 -- IN_Job_18/RConn1
  IN_Job/LConn19 -- IN_Job_19/RConn1
  IN_Job/LConn20 -- IN_Job_20/RConn1
  IN_Job/LConn21 -- IN_Job_21/RConn1
  IN_Job/LConn22 -- IN_Job_22/RConn1
  IN_Job/LConn23 -- IN_Job_23/RConn1
  IN_Job/LConn24 -- IN_Job_24/RConn1
  IN_Job/LConn25 -- IN_Job_25/RConn1
  IN_Job/LConn26 -- IN_Job_26/RConn1
  IN_Job/LConn27 -- IN_Job_27/RConn1
  IN_Job/LConn28 -- IN_Job_28/RConn1
  IN_Job/LConn29 -- IN_Job_29/RConn1
  IN_Job/LConn30 -- IN_Job_30/RConn1
  IN_Job/LConn31 -- IN_Job_31/RConn1
  IN_Job/LConn32 -- IN_Job_32/RConn1
  IN_Job/LConn33 -- IN_Job_33/RConn1
  IN_Job/LConn34 -- IN_Job_34/RConn1
  IN_Job/LConn35 -- IN_Job_35/RConn1
  IN_Job/LConn36 -- IN_Job_36/RConn1
  IN_Job/LConn37 -- IN_Job_37/RConn1
  IN_Job/LConn38 -- IN_Job_38/RConn1
  IN_Job/LConn39 -- IN_Job_39/RConn1
  IN_Job/LConn40 -- IN_Job_40/RConn1
  OUT_Job/RConn1 -- OUT_Job_1/RConn1
  OUT_Job/RConn2 -- OUT_Job_2/RConn1
  OUT_Job/RConn3 -- OUT_Job_3/RConn1
  OUT_Job/RConn4 -- OUT_Job_4/RConn1
  OUT_Job/RConn5 -- OUT_Job_5/RConn1
  OUT_Job/RConn6 -- OUT_Job_6/RConn1
  OUT_Job/RConn7 -- OUT_Job_7/RConn1
  OUT_Job/RConn8 -- OUT_Job_8/RConn1
  OUT_Job/RConn9 -- OUT_Job_9/RConn1
  OUT_Job/RConn10 -- OUT_Job_10/RConn1
  OUT_Job/RConn11 -- OUT_Job_11/RConn1
  OUT_Job/RConn12 -- OUT_Job_12/RConn1
  OUT_Job/RConn13 -- OUT_Job_13/RConn1
  OUT_Job/RConn14 -- OUT_Job_14/RConn1
  OUT_Job/RConn15 -- OUT_Job_15/RConn1
  OUT_Job/RConn16 -- OUT_Job_16/RConn1
  OUT_Job/RConn17 -- OUT_Job_17/RConn1
  OUT_Job/RConn18 -- OUT_Job_18/RConn1
  OUT_Job/RConn19 -- OUT_Job_19/RConn1
  OUT_Job/RConn20 -- OUT_Job_20/RConn1
  OUT_Job/RConn21 -- OUT_Job_21/RConn1
  OUT_Job/RConn22 -- OUT_Job_22/RConn1
  OUT_Job/RConn23 -- OUT_Job_23/RConn1
  OUT_Job/RConn24 -- OUT_Job_24/RConn1
  OUT_Job/RConn25 -- OUT_Job_25/RConn1
  OUT_Job/RConn26 -- OUT_Job_26/RConn1
  OUT_Job/RConn27 -- OUT_Job_27/RConn1
  OUT_Job/RConn28 -- OUT_Job_28/RConn1
  OUT_Job/RConn29 -- OUT_Job_29/RConn1
  OUT_Job/RConn30 -- OUT_Job_30/RConn1
  OUT_Job/RConn31 -- OUT_Job_31/RConn1
  OUT_Job/RConn32 -- OUT_Job_32/RConn1
  OUT_Job/RConn33 -- OUT_Job_33/RConn1
  OUT_Job/RConn34 -- OUT_Job_34/RConn1
  OUT_Job/RConn35 -- OUT_Job_35/RConn1
  OUT_Job/RConn36 -- OUT_Job_36/RConn1
  OUT_Job/RConn37 -- OUT_Job_37/RConn1
  OUT_Job/RConn38 -- OUT_Job_38/RConn1
  OUT_Job/RConn39 -- OUT_Job_39/RConn1
  OUT_Job/RConn40 -- OUT_Job_40/RConn1
  OUT_Job/RConn41 -- OUT_Job_41/RConn1
  OUT_Job/RConn42 -- OUT_Job_42/RConn1

== system ProcessNetworkSimulation/Process_44 ==
  IN_Job : PathCombiner  NumberInputPorts=41
  OUT_Job : OutputSwitch  NumberOutputPorts=45  SwitchingCriterion=From attribute  AttributeName=outputFlowNode
  Process : Subsystem
  IN_Job_1 : PMIOPort  Port=1  Side=Left
  IN_Job_2 : PMIOPort  Port=2  Side=Left
  IN_Job_3 : PMIOPort  Port=3  Side=Left
  IN_Job_4 : PMIOPort  Port=4  Side=Left
  IN_Job_5 : PMIOPort  Port=5  Side=Left
  IN_Job_6 : PMIOPort  Port=6  Side=Left
  IN_Job_7 : PMIOPort  Port=7  Side=Left
  IN_Job_8 : PMIOPort  Port=8  Side=Left
  IN_Job_9 : PMIOPort  Port=9  Side=Left
  IN_Job_10 : PMIOPort  Port=10  Side=Left
  IN_Job_11 : PMIOPort  Port=11  Side=Left
  IN_Job_12 : PMIOPort  Port=12  Side=Left
  IN_Job_13 : PMIOPort  Port=13  Side=Left
  IN_Job_14 : PMIOPort  Port=14  Side=Left
  IN_Job_15 : PMIOPort  Port=15  Side=Left
  IN_Job_16 : PMIOPort  Port=16  Side=Left
  IN_Job_17 : PMIOPort  Port=17  Side=Left
  IN_Job_18 : PMIOPort  Port=18  Side=Left
  IN_Job_19 : PMIOPort  Port=19  Side=Left
  IN_Job_20 : PMIOPort  Port=20  Side=Left
  IN_Job_21 : PMIOPort  Port=21  Side=Left
  IN_Job_22 : PMIOPort  Port=22  Side=Left
  IN_Job_23 : PMIOPort  Port=23  Side=Left
  IN_Job_24 : PMIOPort  Port=24  Side=Left
  IN_Job_25 : PMIOPort  Port=25  Side=Left
  IN_Job_26 : PMIOPort  Port=26  Side=Left
  IN_Job_27 : PMIOPort  Port=27  Side=Left
  IN_Job_28 : PMIOPort  Port=28  Side=Left
  IN_Job_29 : PMIOPort  Port=29  Side=Left
  IN_Job_30 : PMIOPort  Port=30  Side=Left
  IN_Job_31 : PMIOPort  Port=31  Side=Left
  IN_Job_32 : PMIOPort  Port=32  Side=Left
  IN_Job_33 : PMIOPort  Port=33  Side=Left
  IN_Job_34 : PMIOPort  Port=34  Side=Left
  IN_Job_35 : PMIOPort  Port=35  Side=Left
  IN_Job_36 : PMIOPort  Port=36  Side=Left
  IN_Job_37 : PMIOPort  Port=37  Side=Left
  IN_Job_38 : PMIOPort  Port=38  Side=Left
  IN_Job_39 : PMIOPort  Port=39  Side=Left
  IN_Job_40 : PMIOPort  Port=40  Side=Left
  IN_Job_41 : PMIOPort  Port=41  Side=Left
  OUT_Job_1 : PMIOPort  Port=42  Side=Right
  OUT_Job_2 : PMIOPort  Port=43  Side=Right
  OUT_Job_3 : PMIOPort  Port=44  Side=Right
  OUT_Job_4 : PMIOPort  Port=45  Side=Right
  OUT_Job_5 : PMIOPort  Port=46  Side=Right
  OUT_Job_6 : PMIOPort  Port=47  Side=Right
  OUT_Job_7 : PMIOPort  Port=48  Side=Right
  OUT_Job_8 : PMIOPort  Port=49  Side=Right
  OUT_Job_9 : PMIOPort  Port=50  Side=Right
  OUT_Job_10 : PMIOPort  Port=51  Side=Right
  OUT_Job_11 : PMIOPort  Port=52  Side=Right
  OUT_Job_12 : PMIOPort  Port=53  Side=Right
  OUT_Job_13 : PMIOPort  Port=54  Side=Right
  OUT_Job_14 : PMIOPort  Port=55  Side=Right
  OUT_Job_15 : PMIOPort  Port=56  Side=Right
  OUT_Job_16 : PMIOPort  Port=57  Side=Right
  OUT_Job_17 : PMIOPort  Port=58  Side=Right
  OUT_Job_18 : PMIOPort  Port=59  Side=Right
  OUT_Job_19 : PMIOPort  Port=60  Side=Right
  OUT_Job_20 : PMIOPort  Port=61  Side=Right
  OUT_Job_21 : PMIOPort  Port=62  Side=Right
  OUT_Job_22 : PMIOPort  Port=63  Side=Right
  OUT_Job_23 : PMIOPort  Port=64  Side=Right
  OUT_Job_24 : PMIOPort  Port=65  Side=Right
  OUT_Job_25 : PMIOPort  Port=66  Side=Right
  OUT_Job_26 : PMIOPort  Port=67  Side=Right
  OUT_Job_27 : PMIOPort  Port=68  Side=Right
  OUT_Job_28 : PMIOPort  Port=69  Side=Right
  OUT_Job_29 : PMIOPort  Port=70  Side=Right
  OUT_Job_30 : PMIOPort  Port=71  Side=Right
  OUT_Job_31 : PMIOPort  Port=72  Side=Right
  OUT_Job_32 : PMIOPort  Port=73  Side=Right
  OUT_Job_33 : PMIOPort  Port=74  Side=Right
  OUT_Job_34 : PMIOPort  Port=75  Side=Right
  OUT_Job_35 : PMIOPort  Port=76  Side=Right
  OUT_Job_36 : PMIOPort  Port=77  Side=Right
  OUT_Job_37 : PMIOPort  Port=78  Side=Right
  OUT_Job_38 : PMIOPort  Port=79  Side=Right
  OUT_Job_39 : PMIOPort  Port=80  Side=Right
  OUT_Job_40 : PMIOPort  Port=81  Side=Right
  OUT_Job_41 : PMIOPort  Port=82  Side=Right
  OUT_Job_42 : PMIOPort  Port=83  Side=Right
  OUT_Job_43 : PMIOPort  Port=84  Side=Right
  OUT_Job_44 : PMIOPort  Port=85  Side=Right
  OUT_Job_45 : PMIOPort  Port=86  Side=Right
  connections:
  OUT_Job/LConn1 -- Process/RConn1
  IN_Job/RConn1 -- Process/LConn1
  IN_Job/LConn1 -- IN_Job_1/RConn1
  IN_Job/LConn2 -- IN_Job_2/RConn1
  IN_Job/LConn3 -- IN_Job_3/RConn1
  IN_Job/LConn4 -- IN_Job_4/RConn1
  IN_Job/LConn5 -- IN_Job_5/RConn1
  IN_Job/LConn6 -- IN_Job_6/RConn1
  IN_Job/LConn7 -- IN_Job_7/RConn1
  IN_Job/LConn8 -- IN_Job_8/RConn1
  IN_Job/LConn9 -- IN_Job_9/RConn1
  IN_Job/LConn10 -- IN_Job_10/RConn1
  IN_Job/LConn11 -- IN_Job_11/RConn1
  IN_Job/LConn12 -- IN_Job_12/RConn1
  IN_Job/LConn13 -- IN_Job_13/RConn1
  IN_Job/LConn14 -- IN_Job_14/RConn1
  IN_Job/LConn15 -- IN_Job_15/RConn1
  IN_Job/LConn16 -- IN_Job_16/RConn1
  IN_Job/LConn17 -- IN_Job_17/RConn1
  IN_Job/LConn18 -- IN_Job_18/RConn1
  IN_Job/LConn19 -- IN_Job_19/RConn1
  IN_Job/LConn20 -- IN_Job_20/RConn1
  IN_Job/LConn21 -- IN_Job_21/RConn1
  IN_Job/LConn22 -- IN_Job_22/RConn1
  IN_Job/LConn23 -- IN_Job_23/RConn1
  IN_Job/LConn24 -- IN_Job_24/RConn1
  IN_Job/LConn25 -- IN_Job_25/RConn1
  IN_Job/LConn26 -- IN_Job_26/RConn1
  IN_Job/LConn27 -- IN_Job_27/RConn1
  IN_Job/LConn28 -- IN_Job_28/RConn1
  IN_Job/LConn29 -- IN_Job_29/RConn1
  IN_Job/LConn30 -- IN_Job_30/RConn1
  IN_Job/LConn31 -- IN_Job_31/RConn1
  IN_Job/LConn32 -- IN_Job_32/RConn1
  IN_Job/LConn33 -- IN_Job_33/RConn1
  IN_Job/LConn34 -- IN_Job_34/RConn1
  IN_Job/LConn35 -- IN_Job_35/RConn1
  IN_Job/LConn36 -- IN_Job_36/RConn1
  IN_Job/LConn37 -- IN_Job_37/RConn1
  IN_Job/LConn38 -- IN_Job_38/RConn1
  IN_Job/LConn39 -- IN_Job_39/RConn1
  IN_Job/LConn40 -- IN_Job_40/RConn1
  IN_Job/LConn41 -- IN_Job_41/RConn1
  OUT_Job/RConn1 -- OUT_Job_1/RConn1
  OUT_Job/RConn2 -- OUT_Job_2/RConn1
  OUT_Job/RConn3 -- OUT_Job_3/RConn1
  OUT_Job/RConn4 -- OUT_Job_4/RConn1
  OUT_Job/RConn5 -- OUT_Job_5/RConn1
  OUT_Job/RConn6 -- OUT_Job_6/RConn1
  OUT_Job/RConn7 -- OUT_Job_7/RConn1
  OUT_Job/RConn8 -- OUT_Job_8/RConn1
  OUT_Job/RConn9 -- OUT_Job_9/RConn1
  OUT_Job/RConn10 -- OUT_Job_10/RConn1
  OUT_Job/RConn11 -- OUT_Job_11/RConn1
  OUT_Job/RConn12 -- OUT_Job_12/RConn1
  OUT_Job/RConn13 -- OUT_Job_13/RConn1
  OUT_Job/RConn14 -- OUT_Job_14/RConn1
  OUT_Job/RConn15 -- OUT_Job_15/RConn1
  OUT_Job/RConn16 -- OUT_Job_16/RConn1
  OUT_Job/RConn17 -- OUT_Job_17/RConn1
  OUT_Job/RConn18 -- OUT_Job_18/RConn1
  OUT_Job/RConn19 -- OUT_Job_19/RConn1
  OUT_Job/RConn20 -- OUT_Job_20/RConn1
  OUT_Job/RConn21 -- OUT_Job_21/RConn1
  OUT_Job/RConn22 -- OUT_Job_22/RConn1
  OUT_Job/RConn23 -- OUT_Job_23/RConn1
  OUT_Job/RConn24 -- OUT_Job_24/RConn1
  OUT_Job/RConn25 -- OUT_Job_25/RConn1
  OUT_Job/RConn26 -- OUT_Job_26/RConn1
  OUT_Job/RConn27 -- OUT_Job_27/RConn1
  OUT_Job/RConn28 -- OUT_Job_28/RConn1
  OUT_Job/RConn29 -- OUT_Job_29/RConn1
  OUT_Job/RConn30 -- OUT_Job_30/RConn1
  OUT_Job/RConn31 -- OUT_Job_31/RConn1
  OUT_Job/RConn32 -- OUT_Job_32/RConn1
  OUT_Job/RConn33 -- OUT_Job_33/RConn1
  OUT_Job/RConn34 -- OUT_Job_34/RConn1
  OUT_Job/RConn35 -- OUT_Job_35/RConn1
  OUT_Job/RConn36 -- OUT_Job_36/RConn1
  OUT_Job/RConn37 -- OUT_Job_37/RConn1
  OUT_Job/RConn38 -- OUT_Job_38/RConn1
  OUT_Job/RConn39 -- OUT_Job_39/RConn1
  OUT_Job/RConn40 -- OUT_Job_40/RConn1
  OUT_Job/RConn41 -- OUT_Job_41/RConn1
  OUT_Job/RConn42 -- OUT_Job_42/RConn1
  OUT_Job/RConn43 -- OUT_Job_43/RConn1
  OUT_Job/RConn44 -- OUT_Job_44/RConn1
  OUT_Job/RConn45 -- OUT_Job_45/RConn1

== system ProcessNetworkSimulation/Process_45 ==
  IN_Job : PathCombiner  NumberInputPorts=41
  OUT_Job : OutputSwitch  NumberOutputPorts=35  SwitchingCriterion=From attribute  AttributeName=outputFlowNode
  Process : Subsystem
  IN_Job_1 : PMIOPort  Port=1  Side=Left
  IN_Job_2 : PMIOPort  Port=2  Side=Left
  IN_Job_3 : PMIOPort  Port=3  Side=Left
  IN_Job_4 : PMIOPort  Port=4  Side=Left
  IN_Job_5 : PMIOPort  Port=5  Side=Left
  IN_Job_6 : PMIOPort  Port=6  Side=Left
  IN_Job_7 : PMIOPort  Port=7  Side=Left
  IN_Job_8 : PMIOPort  Port=8  Side=Left
  IN_Job_9 : PMIOPort  Port=9  Side=Left
  IN_Job_10 : PMIOPort  Port=10  Side=Left
  IN_Job_11 : PMIOPort  Port=11  Side=Left
  IN_Job_12 : PMIOPort  Port=12  Side=Left
  IN_Job_13 : PMIOPort  Port=13  Side=Left
  IN_Job_14 : PMIOPort  Port=14  Side=Left
  IN_Job_15 : PMIOPort  Port=15  Side=Left
  IN_Job_16 : PMIOPort  Port=16  Side=Left
  IN_Job_17 : PMIOPort  Port=17  Side=Left
  IN_Job_18 : PMIOPort  Port=18  Side=Left
  IN_Job_19 : PMIOPort  Port=19  Side=Left
  IN_Job_20 : PMIOPort  Port=20  Side=Left
  IN_Job_21 : PMIOPort  Port=21  Side=Left
  IN_Job_22 : PMIOPort  Port=22  Side=Left
  IN_Job_23 : PMIOPort  Port=23  Side=Left
  IN_Job_24 : PMIOPort  Port=24  Side=Left
  IN_Job_25 : PMIOPort  Port=25  Side=Left
  IN_Job_26 : PMIOPort  Port=26  Side=Left
  IN_Job_27 : PMIOPort  Port=27  Side=Left
  IN_Job_28 : PMIOPort  Port=28  Side=Left
  IN_Job_29 : PMIOPort  Port=29  Side=Left
  IN_Job_30 : PMIOPort  Port=30  Side=Left
  IN_Job_31 : PMIOPort  Port=31  Side=Left
  IN_Job_32 : PMIOPort  Port=32  Side=Left
  IN_Job_33 : PMIOPort  Port=33  Side=Left
  IN_Job_34 : PMIOPort  Port=34  Side=Left
  IN_Job_35 : PMIOPort  Port=35  Side=Left
  IN_Job_36 : PMIOPort  Port=36  Side=Left
  IN_Job_37 : PMIOPort  Port=37  Side=Left
  IN_Job_38 : PMIOPort  Port=38  Side=Left
  IN_Job_39 : PMIOPort  Port=39  Side=Left
  IN_Job_40 : PMIOPort  Port=40  Side=Left
  IN_Job_41 : PMIOPort  Port=41  Side=Left
  OUT_Job_1 : PMIOPort  Port=42  Side=Right
  OUT_Job_2 : PMIOPort  Port=43  Side=Right
  OUT_Job_3 : PMIOPort  Port=44  Side=Right
  OUT_Job_4 : PMIOPort  Port=45  Side=Right
  OUT_Job_5 : PMIOPort  Port=46  Side=Right
  OUT_Job_6 : PMIOPort  Port=47  Side=Right
  OUT_Job_7 : PMIOPort  Port=48  Side=Right
  OUT_Job_8 : PMIOPort  Port=49  Side=Right
  OUT_Job_9 : PMIOPort  Port=50  Side=Right
  OUT_Job_10 : PMIOPort  Port=51  Side=Right
  OUT_Job_11 : PMIOPort  Port=52  Side=Right
  OUT_Job_12 : PMIOPort  Port=53  Side=Right
  OUT_Job_13 : PMIOPort  Port=54  Side=Right
  OUT_Job_14 : PMIOPort  Port=55  Side=Right
  OUT_Job_15 : PMIOPort  Port=56  Side=Right
  OUT_Job_16 : PMIOPort  Port=57  Side=Right
  OUT_Job_17 : PMIOPort  Port=58  Side=Right
  OUT_Job_18 : PMIOPort  Port=59  Side=Right
  OUT_Job_19 : PMIOPort  Port=60  Side=Right
  OUT_Job_20 : PMIOPort  Port=61  Side=Right
  OUT_Job_21 : PMIOPort  Port=62  Side=Right
  OUT_Job_22 : PMIOPort  Port=63  Side=Right
  OUT_Job_23 : PMIOPort  Port=64  Side=Right
  OUT_Job_24 : PMIOPort  Port=65  Side=Right
  OUT_Job_25 : PMIOPort  Port=66  Side=Right
  OUT_Job_26 : PMIOPort  Port=67  Side=Right
  OUT_Job_27 : PMIOPort  Port=68  Side=Right
  OUT_Job_28 : PMIOPort  Port=69  Side=Right
  OUT_Job_29 : PMIOPort  Port=70  Side=Right
  OUT_Job_30 : PMIOPort  Port=71  Side=Right
  OUT_Job_31 : PMIOPort  Port=72  Side=Right
  OUT_Job_32 : PMIOPort  Port=73  Side=Right
  OUT_Job_33 : PMIOPort  Port=74  Side=Right
  OUT_Job_34 : PMIOPort  Port=75  Side=Right
  OUT_Job_35 : PMIOPort  Port=76  Side=Right
  connections:
  OUT_Job/LConn1 -- Process/RConn1
  IN_Job/RConn1 -- Process/LConn1
  IN_Job/LConn1 -- IN_Job_1/RConn1
  IN_Job/LConn2 -- IN_Job_2/RConn1
  IN_Job/LConn3 -- IN_Job_3/RConn1
  IN_Job/LConn4 -- IN_Job_4/RConn1
  IN_Job/LConn5 -- IN_Job_5/RConn1
  IN_Job/LConn6 -- IN_Job_6/RConn1
  IN_Job/LConn7 -- IN_Job_7/RConn1
  IN_Job/LConn8 -- IN_Job_8/RConn1
  IN_Job/LConn9 -- IN_Job_9/RConn1
  IN_Job/LConn10 -- IN_Job_10/RConn1
  IN_Job/LConn11 -- IN_Job_11/RConn1
  IN_Job/LConn12 -- IN_Job_12/RConn1
  IN_Job/LConn13 -- IN_Job_13/RConn1
  IN_Job/LConn14 -- IN_Job_14/RConn1
  IN_Job/LConn15 -- IN_Job_15/RConn1
  IN_Job/LConn16 -- IN_Job_16/RConn1
  IN_Job/LConn17 -- IN_Job_17/RConn1
  IN_Job/LConn18 -- IN_Job_18/RConn1
  IN_Job/LConn19 -- IN_Job_19/RConn1
  IN_Job/LConn20 -- IN_Job_20/RConn1
  IN_Job/LConn21 -- IN_Job_21/RConn1
  IN_Job/LConn22 -- IN_Job_22/RConn1
  IN_Job/LConn23 -- IN_Job_23/RConn1
  IN_Job/LConn24 -- IN_Job_24/RConn1
  IN_Job/LConn25 -- IN_Job_25/RConn1
  IN_Job/LConn26 -- IN_Job_26/RConn1
  IN_Job/LConn27 -- IN_Job_27/RConn1
  IN_Job/LConn28 -- IN_Job_28/RConn1
  IN_Job/LConn29 -- IN_Job_29/RConn1
  IN_Job/LConn30 -- IN_Job_30/RConn1
  IN_Job/LConn31 -- IN_Job_31/RConn1
  IN_Job/LConn32 -- IN_Job_32/RConn1
  IN_Job/LConn33 -- IN_Job_33/RConn1
  IN_Job/LConn34 -- IN_Job_34/RConn1
  IN_Job/LConn35 -- IN_Job_35/RConn1
  IN_Job/LConn36 -- IN_Job_36/RConn1
  IN_Job/LConn37 -- IN_Job_37/RConn1
  IN_Job/LConn38 -- IN_Job_38/RConn1
  IN_Job/LConn39 -- IN_Job_39/RConn1
  IN_Job/LConn40 -- IN_Job_40/RConn1
  IN_Job/LConn41 -- IN_Job_41/RConn1
  OUT_Job/RConn1 -- OUT_Job_1/RConn1
  OUT_Job/RConn2 -- OUT_Job_2/RConn1
  OUT_Job/RConn3 -- OUT_Job_3/RConn1
  OUT_Job/RConn4 -- OUT_Job_4/RConn1
  OUT_Job/RConn5 -- OUT_Job_5/RConn1
  OUT_Job/RConn6 -- OUT_Job_6/RConn1
  OUT_Job/RConn7 -- OUT_Job_7/RConn1
  OUT_Job/RConn8 -- OUT_Job_8/RConn1
  OUT_Job/RConn9 -- OUT_Job_9/RConn1
  OUT_Job/RConn10 -- OUT_Job_10/RConn1
  OUT_Job/RConn11 -- OUT_Job_11/RConn1
  OUT_Job/RConn12 -- OUT_Job_12/RConn1
  OUT_Job/RConn13 -- OUT_Job_13/RConn1
  OUT_Job/RConn14 -- OUT_Job_14/RConn1
  OUT_Job/RConn15 -- OUT_Job_15/RConn1
  OUT_Job/RConn16 -- OUT_Job_16/RConn1
  OUT_Job/RConn17 -- OUT_Job_17/RConn1
  OUT_Job/RConn18 -- OUT_Job_18/RConn1
  OUT_Job/RConn19 -- OUT_Job_19/RConn1
  OUT_Job/RConn20 -- OUT_Job_20/RConn1
  OUT_Job/RConn21 -- OUT_Job_21/RConn1
  OUT_Job/RConn22 -- OUT_Job_22/RConn1
  OUT_Job/RConn23 -- OUT_Job_23/RConn1
  OUT_Job/RConn24 -- OUT_Job_24/RConn1
  OUT_Job/RConn25 -- OUT_Job_25/RConn1
  OUT_Job/RConn26 -- OUT_Job_26/RConn1
  OUT_Job/RConn27 -- OUT_Job_27/RConn1
  OUT_Job/RConn28 -- OUT_Job_28/RConn1
  OUT_Job/RConn29 -- OUT_Job_29/RConn1
  OUT_Job/RConn30 -- OUT_Job_30/RConn1
  OUT_Job/RConn31 -- OUT_Job_31/RConn1
  OUT_Job/RConn32 -- OUT_Job_32/RConn1
  OUT_Job/RConn33 -- OUT_Job_33/RConn1
  OUT_Job/RConn34 -- OUT_Job_34/RConn1
  OUT_Job/RConn35 -- OUT_Job_35/RConn1
